simulink model "Planta"  (R2017a)
settings: Solver=VariableStepAuto  StartTime=0.0  StopTime=100.0  RelTol=1e-3
values from neighbouring files (symbols this model uses):
  b_h = b_eq_h * r_h ^ 2 / R_d ^ 2    (= 28800)    [automatas_matlab.m]
  b_t = b_eq_t * r_t ^ 2 / R_w_t ^ 2    (= 27000)    [automatas_matlab.m]
  b_w_h = 30000    [automatas_matlab.m]
  g = 9.80665    [automatas_matlab.m]
  h_contenedor = 2.79    [automatas_matlab.m]
  K_w_h = 1800000    [automatas_matlab.m]
  M_h = (J_d + J_m_h * r_h ^ 2)/ R_d ^ 2    (= 48014.2222222)    [automatas_matlab.m]
  m_l = 65000    [automatas_matlab.m]
  M_t = m_c + (J_w_t + J_m_t * r_t ^ 2)/ R_w_t ^ 2    (= 59008)    [automatas_matlab.m]
  R_d = 0.75    [automatas_matlab.m]
  r_h = 30    [automatas_matlab.m]
  r_t = 15    [automatas_matlab.m]
  R_w_t = 0.5    [automatas_matlab.m]
  x_t0 = 0    [automatas_matlab.m]
  y_t0 = 45    [automatas_matlab.m]    (also in crane.m; plot_crane.m; plot_crane_test.m)
  yl0 = h_contenedor + 5    (= 7.79)    [automatas_matlab.m]
settings Model: Creator=laure  LastModifiedBy=laure

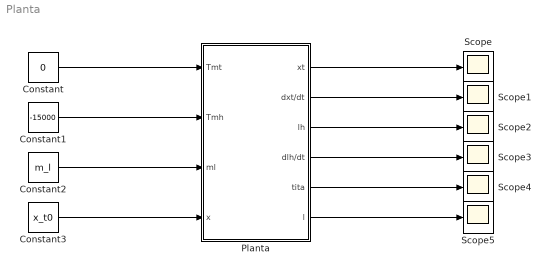
== system Planta ==
  Constant : Constant  Value=0
  Constant1 : Constant  Value=-15000
  Constant2 : Constant  Value=m_l
  Constant3 : Constant  Value=x_t0
  Planta : Subsystem
  Scope{,1..5} (6 alike) : Scope
  wires:
  Planta/1(xt) -> Scope/1
  Planta/2(dxt/dt) -> Scope1/1
  Planta/3(lh) -> Scope2/1
  Planta/4(dlh/dt) -> Scope3/1
  Planta/5(tita) -> Scope4/1
  Planta/6(l) -> Scope5/1
  Constant/1 -> Planta/1(Tmt)
  Constant1/1 -> Planta/2(Tmh)
  Constant2/1 -> Planta/3(ml)
  Constant3/1 -> Planta/4(x)

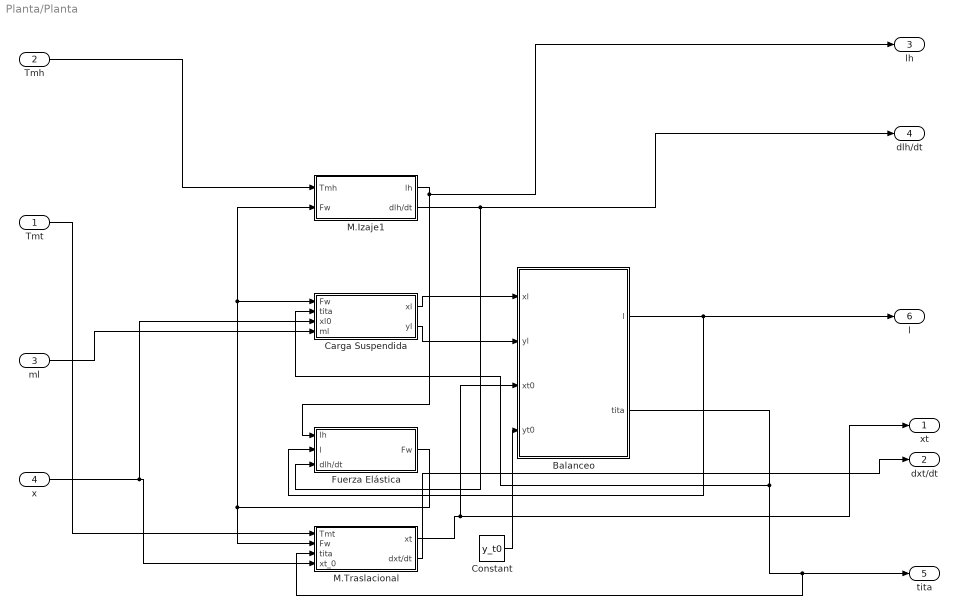
== system Planta/Planta ==
  Tmt : Inport
  Tmh : Inport  Port=2
  ml : Inport  Port=3
  x : Inport  Port=4
  Balanceo : MATLAB Function  TreatAsAtomicUnit=on
  Carga Suspendida : Subsystem
  Constant : Constant  Value=y_t0
  Fuerza Elástica : Subsystem
  M.Izaje1 : Subsystem
  M.Traslacional : Subsystem
  xt : Outport
  dxt/dt : Outport  Port=2
  lh : Outport  Port=3
  dlh/dt : Outport  Port=4
  tita : Outport  Port=5
  l : Outport  Port=6
  wires:
  Balanceo/2(tita) -> Carga Suspendida/2(tita), M.Traslacional/3(tita), tita/1
  Balanceo/1(l) -> Fuerza Elástica/2(l), l/1
  M.Izaje1/2(dlh/dt) -> Fuerza Elástica/3(dlh/dt), dlh/dt/1
  Fuerza Elástica/1(Fw) -> M.Traslacional/2(Fw), Carga Suspendida/1(Fw), M.Izaje1/2(Fw)
  x/1 -> Carga Suspendida/3(xl0), M.Traslacional/4(xt_0)
  ml/1 -> Carga Suspendida/4(ml)
  M.Izaje1/1(lh) -> lh/1, Fuerza Elástica/1(lh)
  Tmh/1 -> M.Izaje1/1(Tmh)
  Tmt/1 -> M.Traslacional/1("Tmt ")
  Carga Suspendida/1(xl) -> Balanceo/1(xl)
  Carga Suspendida/2(yl) -> Balanceo/2(yl)
  M.Traslacional/1(xt) -> Balanceo/3(xt0), xt/1
  M.Traslacional/2(dxt/dt) -> dxt/dt/1
  Constant/1 -> Balanceo/4(yt0)

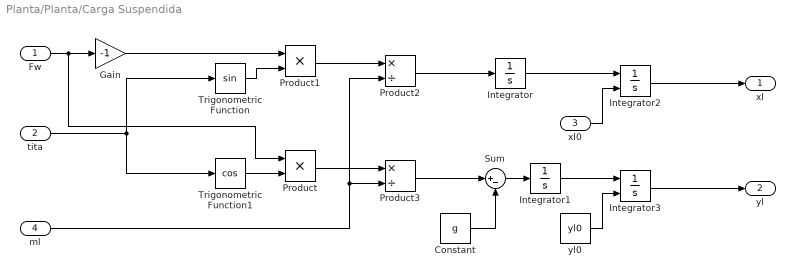
== system Planta/Planta/Carga Suspendida ==
  Fw : Inport
  tita : Inport  Port=2
  xl0 : Inport  Port=3
  ml : Inport  Port=4
  Constant : Constant  Value=g
  Gain : Gain  Gain=-1
  Integrator : Integrator
  Integrator1 : Integrator
  Integrator2 : Integrator  InitialConditionSource=external
  Integrator3 : Integrator  InitialConditionSource=external
  Product : Product
  Product1 : Product
  Product2 : Product  Inputs=*/
  Product3 : Product  Inputs=*/
  Sum : Sum  Inputs=|+-
  Trigonometric Function : Trigonometry
  Trigonometric Function1 : Trigonometry  Operator=cos
  yl0 : Constant  Value=yl0
  xl : Outport
  yl : Outport  Port=2
  wires:
  tita/1 -> Trigonometric Function/1, Trigonometric Function1/1
  Constant/1 -> Sum/2
  Trigonometric Function1/1 -> Product/2
  Fw/1 -> Product/1, Gain/1
  Trigonometric Function/1 -> Product1/2
  Sum/1 -> Integrator1/1
  Integrator/1 -> Integrator2/1
  Integrator1/1 -> Integrator3/1
  yl0/1 -> Integrator3/2
  xl0/1 -> Integrator2/2
  Integrator2/1 -> xl/1
  Integrator3/1 -> yl/1
  Product/1 -> Product3/1
  Product1/1 -> Product2/1
  ml/1 -> Product2/2, Product3/2
  Product2/1 -> Integrator/1
  Product3/1 -> Sum/1
  Gain/1 -> Product1/1

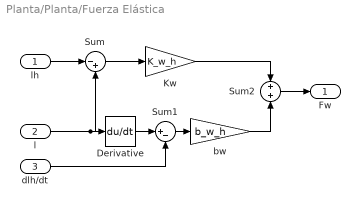
== system Planta/Planta/Fuerza Elástica ==
  lh : Inport
  l : Inport  Port=2
  dlh/dt : Inport  Port=3
  Derivative : Derivative
  Kw : Gain  Gain=K_w_h
  Sum : Sum  Inputs=|-+
  Sum1 : Sum  Inputs=|+-
  Sum2 : Sum
  bw : Gain  Gain=b_w_h
  Fw : Outport
  wires:
  l/1 -> Sum/2, Derivative/1
  lh/1 -> Sum/1
  Sum/1 -> Kw/1
  Derivative/1 -> Sum1/1
  dlh/dt/1 -> Sum1/2
  Sum1/1 -> bw/1
  Sum2/1 -> Fw/1
  Kw/1 -> Sum2/1
  bw/1 -> Sum2/2

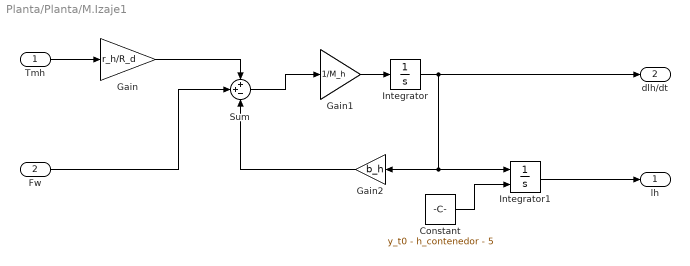
== system Planta/Planta/M.Izaje1 ==
  Tmh : Inport
  Fw : Inport  Port=2
  Constant : Constant  Value=y_t0 - h_contenedor - 5
  Gain : Gain  Gain=r_h/R_d
  Gain1 : Gain  Gain=1/M_h
  Gain2 : Gain  Gain=b_h
  Integrator : Integrator
  Integrator1 : Integrator  InitialConditionSource=external
  Sum : Sum  Inputs=++-
  lh : Outport
  dlh/dt : Outport  Port=2
  wires:
  Tmh/1 -> Gain/1
  Gain/1 -> Sum/1
  Sum/1 -> Gain1/1
  Gain1/1 -> Integrator/1
  Integrator/1 -> dlh/dt/1, Integrator1/1, Gain2/1
  Gain2/1 -> Sum/3
  Fw/1 -> Sum/2
  Constant/1 -> Integrator1/2
  Integrator1/1 -> lh/1

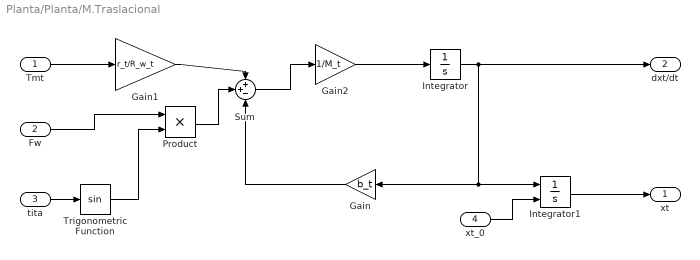
== system Planta/Planta/M.Traslacional ==
  "Tmt " : Inport
  Fw : Inport  Port=2
  tita : Inport  Port=3
  xt_0 : Inport  Port=4
  Gain : Gain  Gain=b_t
  Gain1 : Gain  Gain=r_t/R_w_t
  Gain2 : Gain  Gain=1/M_t
  Integrator : Integrator
  Integrator1 : Integrator  InitialConditionSource=external
  Product : Product
  Sum : Sum  Inputs=++-
  Trigonometric Function : Trigonometry
  xt : Outport
  dxt/dt : Outport  Port=2
  wires:
  Gain2/1 -> Integrator/1
  Trigonometric Function/1 -> Product/2
  tita/1 -> Trigonometric Function/1
  Integrator/1 -> dxt/dt/1, Integrator1/1, Gain/1
  Gain/1 -> Sum/3
  Fw/1 -> Product/1
  Product/1 -> Sum/2
  Sum/1 -> Gain2/1
  Gain1/1 -> Sum/1
  xt_0/1 -> Integrator1/2
  "Tmt "/1 -> Gain1/1
  Integrator1/1 -> xt/1

== matlab function Planta/Balanceo ==
  data: xl input; l output; yl input; xt0 input; yt0 input; tita output
function [l,tita] = fcn(xl,yl,xt0,yt0)

deltax = (xl - xt0);
deltay = -(yl - yt0);


l = sqrt((deltax ^ 2) + (deltay ^ 2));

tita = atan2(deltax, deltay);

end
